simulink model "test2"  (Simulink 7.5)
settings: Solver=ode45  StartTime=0.0  StopTime=10.0  RelTol=1e-3
InitFcn:
  | %% DSPBuilder Start
  | alt_dspbuilder_update_model(bdroot)
  | %% DSPBuilder End
libraries: allblocks_alteradspbuilder2 x3
settings Model: Creator=Administrator  LastModifiedBy=Administrator

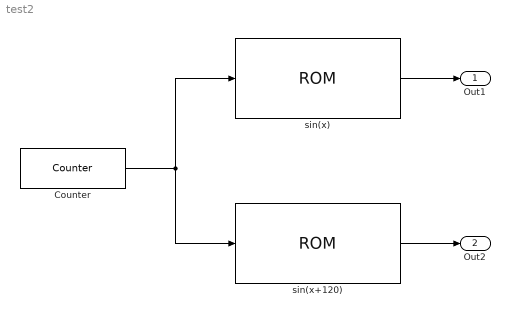
== system test2 ==
  Counter : allblocks_alteradspbuilder2/Counter  BusType=Unsigned Integer  bwl=12  bwr=0  use_modulo=on  modulo=4096  SpecifyClock=off  direction=Increment  use_sload=off  use_sset=off  svalue=1  use_clk_ena=off  use_ena=off  use_sclr=off  pipeline_display=1
  sin(x) : allblocks_alteradspbuilder2/ROM  numwords=4096  BusType=Signed Fractional  bwl=2  bwr=14  memory_type=M9K  ram_type=ROM  initialization=From MATLAB array  init_file=input.hex  init_array=sin([0:2*pi/(2^12):2*pi])  register_outputs=off  use_ena=off  ClockPhase=1  pipeline_display=1  allowFloatingPointOverride=on  logOutputs=off  logFile=C:\altera\13.1\quartus\dsp_builder\tb_test2\test2_sin%28x%29.fixedpointlog  enable_runtime_mod=off  instance_name=AAAA
  sin(x+120) : allblocks_alteradspbuilder2/ROM  numwords=4096  BusType=Signed Fractional  bwl=2  bwr=14  memory_type=M9K  ram_type=ROM  initialization=From MATLAB array  init_file=input.hex  init_array=sin([0:2*pi/(2^12):2*pi]-2*pi/3)  register_outputs=off  use_ena=off  ClockPhase=1  pipeline_display=1  allowFloatingPointOverride=on  logOutputs=off  logFile=C:\altera\13.1\quartus\dsp_builder\tb_test2\test2_sin%28x%2B120%29.fixedpointlog  enable_runtime_mod=off  instance_name=AAAA
  Out1 : Outport  OutDataType=fixdt(1, 16)  OutScaling=2^0
  Out2 : Outport  Port=2  OutDataType=fixdt(1, 16)  OutScaling=2^0
  wires:
  Counter/1 -> sin(x)/1, sin(x+120)/1
  sin(x)/1 -> Out1/1
  sin(x+120)/1 -> Out2/1
